simulink model "lab1_model1"  (R2021b)
settings: Solver=VariableStepAuto  StartTime=0.0  StopTime=60  RelTol=1e-3
libraries: cstblocks x2
settings Model: Creator=2710818Z  LastModifiedBy=12288

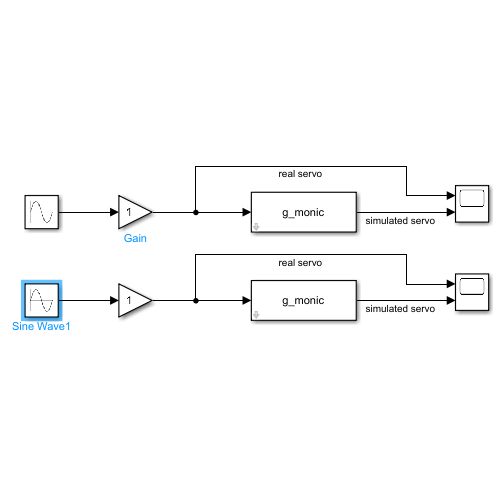
[thumbnail: Simulink's stored preview of the top-level diagram]
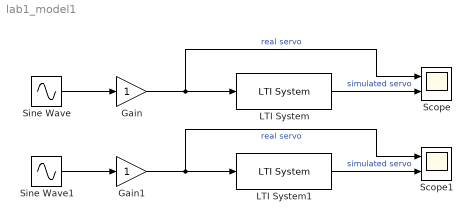
== system lab1_model1 ==
  Gain : Gain
  Gain1 : Gain
  LTI System : cstblocks/LTI System  sys=g_monic  IC=[]
  LTI System1 : cstblocks/LTI System  sys=g_monic  IC=[]
  Scope : Scope  NumInputPorts=2
  Scope1 : Scope  NumInputPorts=2
  Sine Wave : Sin  Phase=pi/2  SampleTime=0
  Sine Wave1 : Sin  Frequency=5  Phase=pi/2  SampleTime=0
  wires:
  Sine Wave/1 -> Gain/1
  Gain/1 -> Scope/1, LTI System/1  "real servo"
  LTI System/1 -> Scope/2  "simulated servo"
  LTI System1/1 -> Scope1/2  "simulated servo"
  Gain1/1 -> Scope1/1, LTI System1/1  "real servo"
  Sine Wave1/1 -> Gain1/1
